simulink model "P1"  (R2024b)
settings: Solver=VariableStepAuto  StartTime=0.0  StopTime=10.0  RelTol=1e-3
settings Model: Creator=PROBOOK  LastModifiedBy=PROBOOK

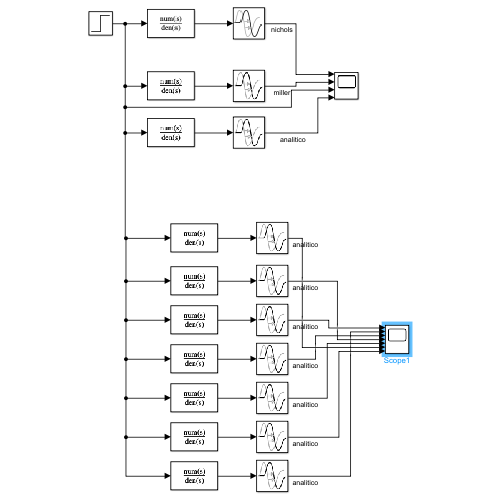
[thumbnail: Simulink's stored preview of the top-level diagram]
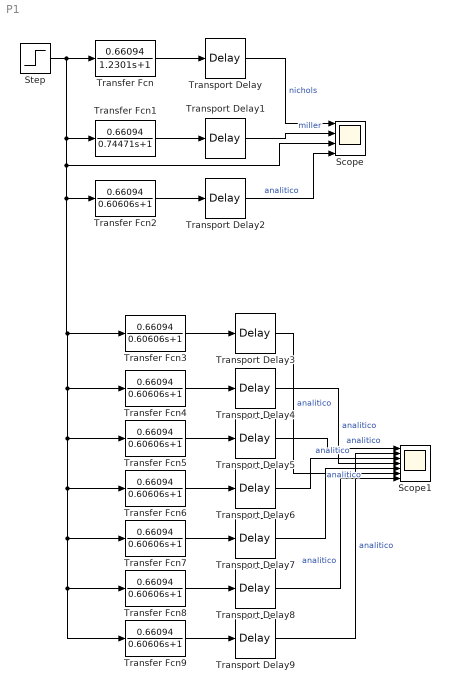
== system P1 ==
  Scope : Scope  NumInputPorts=4
  Scope1 : Scope  NumInputPorts=7
  Step : Step  After=1.5  SampleTime=0
  Transfer Fcn : TransferFcn  Numerator=[0.66094]  Denominator=[1.2301 1]
  Transfer Fcn1 : TransferFcn  Numerator=[0.66094]  Denominator=[0.74471 1]
  Transfer Fcn{2..9} (8 alike) : TransferFcn  Numerator=[0.66094]  Denominator=[0.60606 1]
  Transport Delay : TransportDelay  DelayTime=0.26539
  Transport Delay1 : TransportDelay  DelayTime=0.26539
  Transport Delay2 : TransportDelay  DelayTime=0.40404
  Transport Delay3 : TransportDelay  DelayTime=0
  Transport Delay4 : TransportDelay  DelayTime=0.5
  Transport Delay5 : TransportDelay
  Transport Delay6 : TransportDelay  DelayTime=1.5
  Transport Delay7 : TransportDelay  DelayTime=2
  Transport Delay8 : TransportDelay  DelayTime=2.5
  Transport Delay9 : TransportDelay  DelayTime=3
  wires:
  Transport Delay/1 -> Scope/1  "nichols"
  Transfer Fcn/1 -> Transport Delay/1
  Transfer Fcn1/1 -> Transport Delay1/1
  Step/1 -> Scope/3, Transfer Fcn4/1, Transfer Fcn5/1, Transfer Fcn6/1, Transfer Fcn7/1, Transfer Fcn8/1, Transfer Fcn9/1, Transfer Fcn3/1, Transfer Fcn2/1, Transfer Fcn1/1, Transfer Fcn/1
  Transfer Fcn2/1 -> Transport Delay2/1
  Transport Delay1/1 -> Scope/2  "miller"
  Transport Delay2/1 -> Scope/4  "analitico"
  Transfer Fcn3/1 -> Transport Delay3/1
  Transfer Fcn4/1 -> Transport Delay4/1
  Transfer Fcn5/1 -> Transport Delay5/1
  Transfer Fcn6/1 -> Transport Delay6/1
  Transfer Fcn9/1 -> Transport Delay9/1
  Transfer Fcn8/1 -> Transport Delay8/1
  Transfer Fcn7/1 -> Transport Delay7/1
  Transport Delay9/1 -> Scope1/2  "analitico"
  Transport Delay8/1 -> Scope1/7  "analitico"
  Transport Delay7/1 -> Scope1/5  "analitico"
  Transport Delay6/1 -> Scope1/3  "analitico"
  Transport Delay5/1 -> Scope1/1  "analitico"
  Transport Delay4/1 -> Scope1/4  "analitico"
  Transport Delay3/1 -> Scope1/6  "analitico"
